simulink model "feedback_lin"  (R2023b)
settings: Solver=VariableStepAuto  StartTime=0.0  StopTime=10.0  RelTol=1e-3
values from neighbouring files (symbols this model uses):
  A_ob = A - L*C    [main_feedback_lin.m]
  B_ob = [ B - L*D, L]    [main_feedback_lin.m]
  C_ob = eye(n)    [main_feedback_lin.m]
  D_ob = zeros(n, m+p)    [main_feedback_lin.m]
undefined symbols (not defined in the file or in its folder): x1_eq0, x2_eq0
settings Model: Creator=lollo  LastModifiedBy=lollo

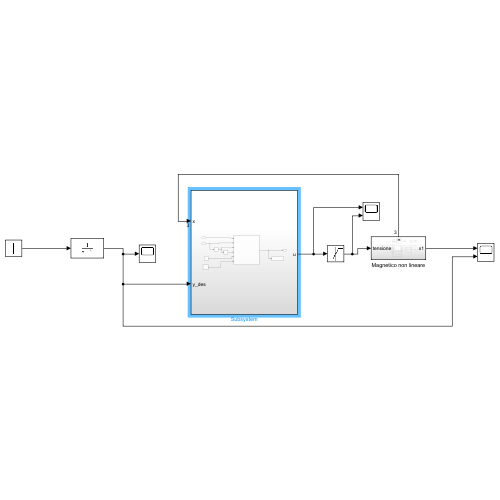
[thumbnail: Simulink's stored preview of the top-level diagram]
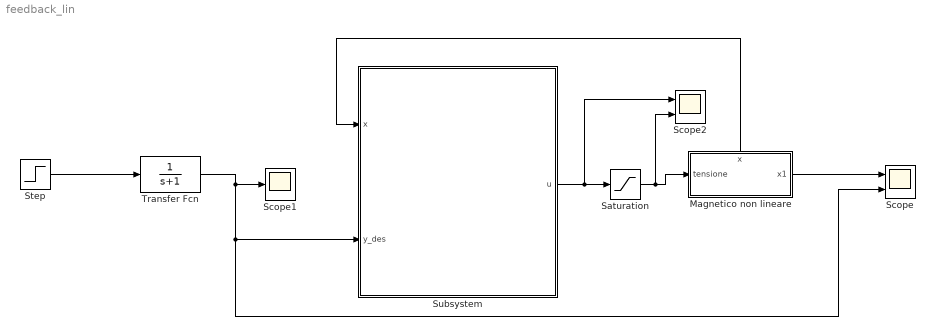
== system feedback_lin ==
  Magnetico non lineare : Subsystem
      settings: PortSchema="{\"entries\":[{\"content\":{\"sides\":[{\"content\":{\"connectorIds\":[\"In1\"]},\"type\":\"ConnectorPlacement.EquallySpacedRectSide\",\"uuid\":\"4c2628b7-19c4-4753-accd-078547eff280\"},{\"content\":{\"connectorIds\":[\"Out1\"],\"side\":\"RIGHT\"},\"type\":\"ConnectorPlacement.EquallySpacedRectSide\",\"uuid\":\"46f8a782-99b4-4db5-ac9e-879226864e1a\"},{\"content\":{\"connectorIds\":[\"Out2\"],\"side\":\"TOP\"},\"type\":\"ConnectorPlacement.EquallySpacedRectSide\",\"uuid\":\"e9ea6a3a-0b10-4f27-be26-5b91ce6de957\"}]},\"type\":\"ConnectorPlacement.EquallySpacedConnector\",\"uuid\":\"8380a659-82e1-48e4-be7e-4b84feeb9f50\"}],\"packageUris\":[\"http://schema.mathworks.com/mf0/Connector/R2020b\"],\"version\":\"1.0\"}"
  Saturation : Saturate  UpperLimit=23  LowerLimit=0
  Scope : Scope  NumInputPorts=2
  Scope1 : Scope
  Scope2 : Scope  NumInputPorts=2
  Step : Step  After=0.001  SampleTime=0
  Subsystem : Subsystem
  Transfer Fcn : TransferFcn  Denominator=[1 1]
  wires:
  Magnetico non lineare/2(x) -> Subsystem/1(x)
  Step/1 -> Transfer Fcn/1
  Magnetico non lineare/1(x1) -> Scope/1
  Transfer Fcn/1 -> Scope1/1, Scope/2, Subsystem/2(y_des)
  Subsystem/1(u) -> Scope2/1, Saturation/1
  Saturation/1 -> Scope2/2, Magnetico non lineare/1(tensione)

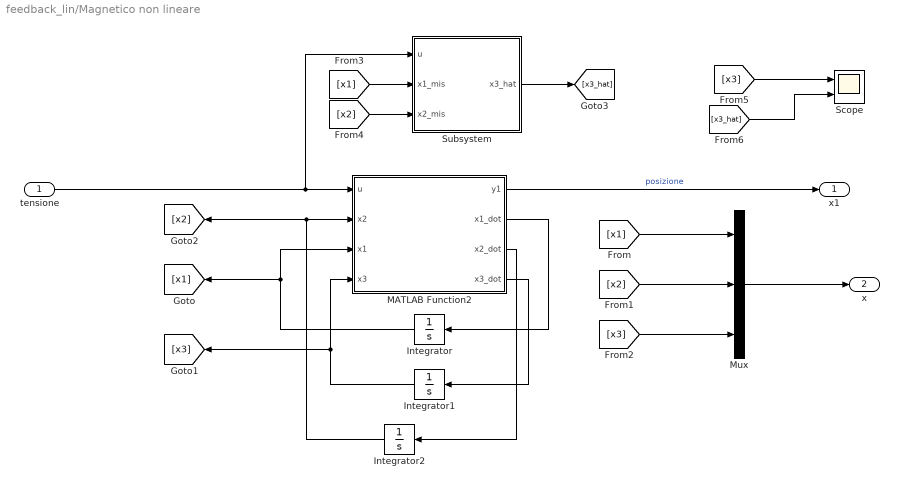
== system feedback_lin/Magnetico non lineare ==
  tensione : Inport
  Integrator : Integrator
  Integrator1 : Integrator
  Integrator2 : Integrator
  MATLAB Function2 : MATLAB Function  TreatAsAtomicUnit=on
  Mux : Mux  Inputs=3
  Scope : Scope  NumInputPorts=2
  Subsystem : Subsystem
  x1 : Outport
  x : Outport  Port=2
  wires:
  tensione/1 -> Subsystem/1(u), MATLAB Function2/1(u)
  MATLAB Function2/1(y1) -> x1/1  "posizione"
  MATLAB Function2/2(x1_dot) -> Integrator/1
  Integrator/1 -> MATLAB Function2/3(x1), [x1]
  MATLAB Function2/4(x3_dot) -> Integrator1/1
  Integrator1/1 -> [x3], MATLAB Function2/4(x3)
  [x1] -> Mux/1
  [x2] -> Mux/2
  [x3] -> Mux/3
  Mux/1 -> x/1
  MATLAB Function2/3(x2_dot) -> Integrator2/1
  [x1] -> Subsystem/2(x1_mis)
  [x2] -> Subsystem/3(x2_mis)
  Subsystem/1(x3_hat) -> [x3_hat]
  [x3_hat] -> Scope/2
  [x3] -> Scope/1
  Integrator2/1 -> MATLAB Function2/2(x2), [x2]

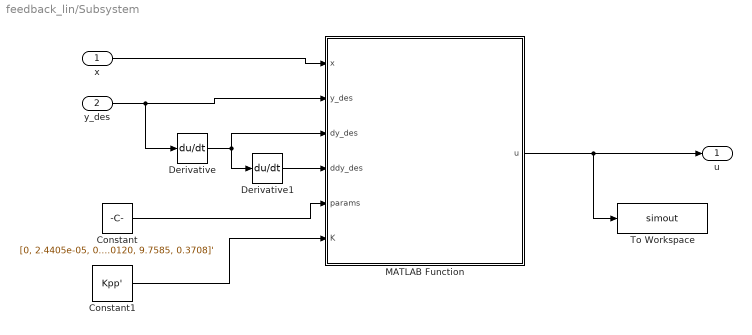
== system feedback_lin/Subsystem ==
  x : Inport
  y_des : Inport  Port=2
  Constant : Constant  Value=[0, 2.4405e-05, 0.0657, 0.0120, 9.7585, 0.3708]'
  Constant1 : Constant  Value=Kpp'
  Derivative : Derivative
  Derivative1 : Derivative
  MATLAB Function : MATLAB Function  TreatAsAtomicUnit=on
  To Workspace : ToWorkspace  VariableName=simout  SaveFormat=Timeseries  SampleTime=-1
  u : Outport
  wires:
  y_des/1 -> Derivative/1, MATLAB Function/2(y_des)
  x/1 -> MATLAB Function/1(x)
  MATLAB Function/1(u) -> To Workspace/1, u/1
  Derivative/1 -> Derivative1/1, MATLAB Function/3(dy_des)
  Constant/1 -> MATLAB Function/5(params)
  Derivative1/1 -> MATLAB Function/4(ddy_des)
  Constant1/1 -> MATLAB Function/6(K)

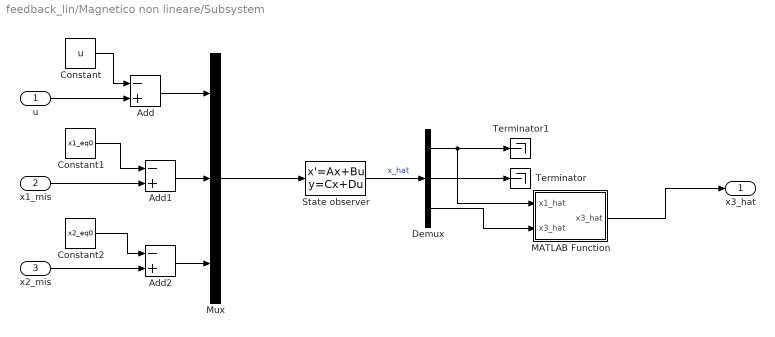
== system feedback_lin/Magnetico non lineare/Subsystem ==
  u : Inport
  x1_mis : Inport  Port=2
  x2_mis : Inport  Port=3
  Add : Sum  Inputs=-+
  Add1 : Sum  Inputs=-+
  Add2 : Sum  Inputs=-+
  Constant : Constant  Value=u
  Constant1 : Constant  Value=x1_eq0
  Constant2 : Constant  Value=x2_eq0
  Demux : Demux  Outputs=3
  MATLAB Function : MATLAB Function  TreatAsAtomicUnit=on
  Mux : Mux  Inputs=3
  State observer : StateSpace  A=A_ob  B=B_ob  C=C_ob  D=D_ob  InitialCondition=[0;0;0]  ParameterTunability=Unconstrained
  Terminator : Terminator
  Terminator1 : Terminator
  x3_hat : Outport
  wires:
  x1_mis/1 -> Add1/2
  u/1 -> Add/2
  Mux/1 -> State observer/1
  State observer/1 -> Demux/1  "x_hat"
  Demux/1 -> MATLAB Function/1(x1_hat), Terminator1/1
  Demux/2 -> Terminator/1
  Constant/1 -> Add/1
  Constant1/1 -> Add1/1
  Constant2/1 -> Add2/1
  x2_mis/1 -> Add2/2
  Add/1 -> Mux/1
  Add1/1 -> Mux/2
  Add2/1 -> Mux/3
  MATLAB Function/1(x3_hat) -> x3_hat/1
  Demux/3 -> MATLAB Function/2("x3_hat ")

== matlab function feedback_lin/Magnetico non lineare/Subsystem/MATLAB Function ==
  data: x1_hat input; x3_hat output; x3_hat input
function x3_hat = fcn(x1_hat, x3_hat)

if x1_hat<=0 && x3_hat<=0
    x3_hat=0;
end

== matlab function feedback_lin/Subsystem/MATLAB Function ==
  data: x input; u output; y_des input; dy_des input; ddy_des input; params input; K input
function u = feedback_linearization_control(x, y_des, dy_des, ddy_des, params, K)
    % Estrai parametri
    k_aero = params(1);
    k_mag  = params(2);
    m      = params(3);
    y0     = params(4);
    Rtot   = params(5);
    Lc     = params(6);
    g      = 9.81;

    % Stati
    x1 = x(1); % posizione
    x2 = x(2); % corrente
    x3 = x(3); % velocità

    % Derivate
    denom = (y0 - x1);
    if denom <= 0
        error('Denominatore nullo o negativo: instabilità elettromagnetica');
    end

    % Calcola seconda derivata (accelerazione)
    xdot3 = (k_aero/m)*x3 + (k_mag/m)*(x2 / denom)^2 - g;

    % Calcola derivata di corrente x2 (richiede input u)
    % da: dx2 = -(Rtot/Lc)*x2 + (1/Lc)*u;
    % => u comparirà nella terza derivata

    % Calcolo della terza derivata (solo parte non u)
    dBdx1 = (2 * k_mag * x2^2) / (m * denom^3);
    dBdx2 = (4 * k_mag * x2) / (m * denom^2);
    dBdx3 = (k_aero/m);

    % Parte non lineare alpha(x)
    alpha = dBdx1 * x3 + dBdx2 * (-(Rtot/Lc)*x2) + dBdx3 * xdot3;

    % Parte moltiplicativa davanti a u (beta(x))
    beta = dBdx2 * (1/Lc);

    % Guadagni desiderati (dati da specifica: esempio polo a - 2, -2, -3)
    
    e = x1 - y_des;
    de = x3 - dy_des;
    dde = xdot3 - ddy_des;
    assignin('base', 'e', e)
    assignin('base', 'ed', de)
    assignin('base', 'edd', dde)

    v = -K' * [e; de; dde];

    % Controllo finale
    u = (1/beta) * (v - alpha);
end

== matlab function feedback_lin/Magnetico non lineare/MATLAB Function2 ==
  data: u input; y1 output; x2 input; x1_dot output; x2_dot output; x1 input; x3 input; x3_dot output
function [y1,x1_dot, x2_dot, x3_dot] = fcn(u, x2, x1, x3)
    m = 0.0657;
    g = 9.81;
    k_mag = 2.4405e-05;
    Rtot = 9.7585;
    Lc = 0.3708;
    y0 = 0.012;
    
    x2_dot = 1/Lc*(-Rtot*x2 + u);

    x1_dot = x3;
    if x1 < y0
        x3_dot = (k_mag/m)*(x2/(y0-x1))^2 - g;
    else
        x1 = 0.012;
        x3_dot = 0;
        x3 = 0;
    end

    
    % condizioni
    if x1 <=0 && x3_dot < 0
        x1 = 0;
        x3 = 0;
        x3_dot = 0;
    end
y1 = x1;
